simulink model "phasemixer"  (R2020a)
settings: Solver=VariableStepAuto  StartTime=0.0  StopTime=10  MaxStep=1e-3  RelTol=1e-3
InitFcn:
  | Fm = 1e9 , Tm = 1/Fm
libraries: simulink x4, msbPllFoundation x1
settings Model: Creator=hassa  LastModifiedBy=hassa

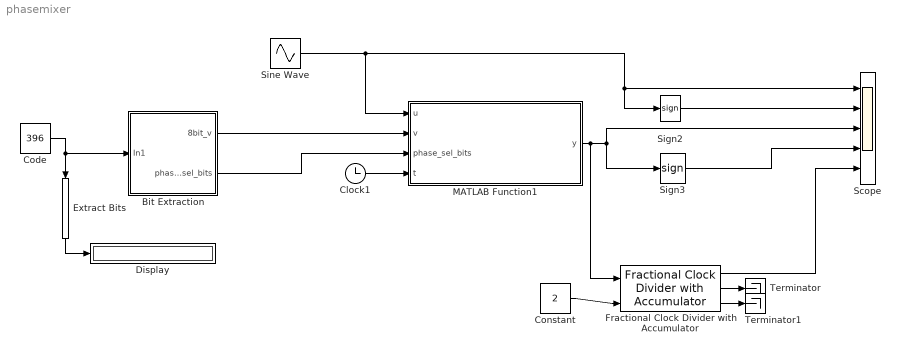
== system phasemixer ==
  Bit Extraction : Subsystem
  Clock1 : Clock
  Code : Constant  Value=396  OutDataTypeStr=uint16
  Constant : Constant  Value=2
  Display : Display
      settings: Format=binary (Stored Integer)
  Extract Bits : simulink/Logic and Bit Operations/Extract Bits  bitsToExtract=Range of bits  numBits=8  bitIdxRange=[0 9]  outScalingMode=Preserve fixed-point scaling
  Fractional Clock Divider with Accumulator : msbPllFoundation/Fractional Clock Divider with Accumulator  ExtraBuffer=on  NBuffer=1
      settings: SourceProductBaseCode=AM
  MATLAB Function1 : MATLAB Function  TreatAsAtomicUnit=on
  Scope : Scope  NumInputPorts=5
  Sign2 : Signum
  Sign3 : Signum
  Sine Wave : Sin  Frequency=2*pi  SampleTime=0
  Terminator : Terminator
  Terminator1 : Terminator
  wires:
  Code/1 -> Bit Extraction/1(In1), Extract Bits/1
  Bit Extraction/1(8bit_v) -> MATLAB Function1/2(v)
  Bit Extraction/2(phase_sel_bits) -> MATLAB Function1/3(phase_sel_bits)
  Clock1/1 -> MATLAB Function1/4(t)
  Sign2/1 -> Scope/2
  Sign3/1 -> Scope/4
  MATLAB Function1/1(y) -> Fractional Clock Divider with Accumulator/1, Scope/3, Sign3/1
  Extract Bits/1 -> Display/1
  Constant/1 -> Fractional Clock Divider with Accumulator/2
  Fractional Clock Divider with Accumulator/1 -> Scope/5
  Fractional Clock Divider with Accumulator/3 -> Terminator1/1
  Fractional Clock Divider with Accumulator/2 -> Terminator/1
  Sine Wave/1 -> MATLAB Function1/1(u), Scope/1, Sign2/1

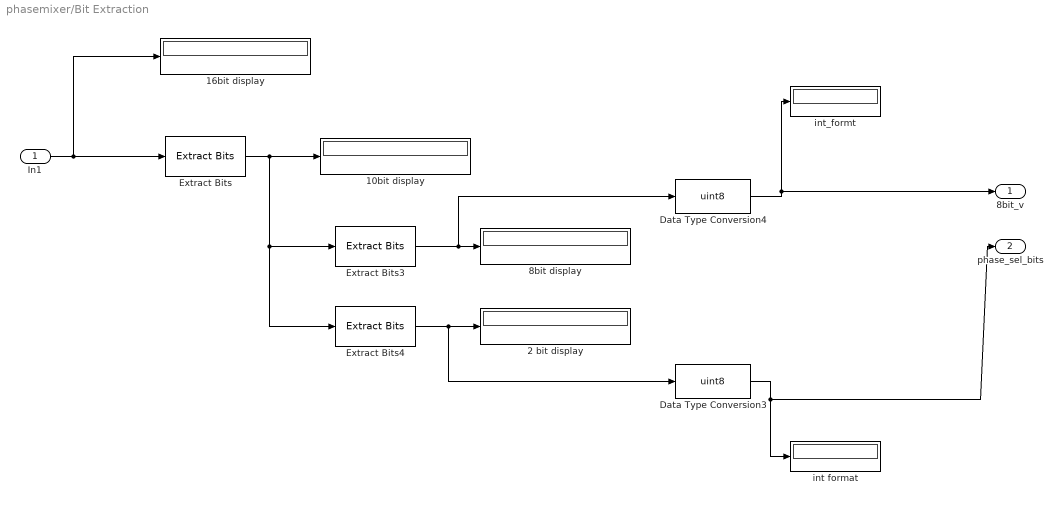
== system phasemixer/Bit Extraction ==
  In1 : Inport
  10bit display : Display
      settings: Format=binary (Stored Integer)
  16bit display : Display
      settings: Format=binary (Stored Integer)
  2 bit display : Display
      settings: Format=binary (Stored Integer)
  8bit display : Display
      settings: Format=binary (Stored Integer)
  Data Type Conversion3 : DataTypeConversion  OutDataTypeStr=uint8
  Data Type Conversion4 : DataTypeConversion  OutDataTypeStr=uint8
  Extract Bits : simulink/Logic and Bit Operations/Extract Bits  bitsToExtract=Range of bits  numBits=8  bitIdxRange=[0 9]  outScalingMode=Preserve fixed-point scaling
  Extract Bits3 : simulink/Logic and Bit Operations/Extract Bits  bitsToExtract=Range of bits  numBits=8  bitIdxRange=[0 7]  outScalingMode=Preserve fixed-point scaling
  Extract Bits4 : simulink/Logic and Bit Operations/Extract Bits  bitsToExtract=Range of bits  numBits=8  bitIdxRange=[8 9]  outScalingMode=Treat bit field as an integer
  int format : Display
  int_formt : Display
  8bit_v : Outport
  phase_sel_bits : Outport  Port=2  VectorParamsAs1DForOutWhenUnconnected=off
  wires:
  In1/1 -> Extract Bits/1, 16bit display/1
  Extract Bits4/1 -> Data Type Conversion3/1, 2 bit display/1
  Extract Bits3/1 -> Data Type Conversion4/1, 8bit display/1
  Extract Bits/1 -> Extract Bits4/1, Extract Bits3/1, 10bit display/1
  Data Type Conversion3/1 -> int format/1, phase_sel_bits/1
  Data Type Conversion4/1 -> 8bit_v/1, int_formt/1

== matlab function phasemixer/MATLAB Function1 ==
  data: u input; y output; v input; phase_sel_bits input; t input
function y  = fcn( u, v, phase_sel_bits, t)

f = 1 ;
% Initialize p1 and p2
p1 = 0.0;
p2 = 0.0;
v1 = double (v)


if phase_sel_bits == 0
    p1 = 0;
    p2 = 90;
elseif phase_sel_bits == 1
    p1 = 90;
    p2 = 180;        
elseif phase_sel_bits == 2
    p1 = 180;
    p2 = 270; 
else
    p1 = 270;
    p2 = 360;    
end

x1 = double(p2*v1)
x2 = double(p1*(255-v1))

inter_pol = (v1/ 255.0) *p2 + ((255.0 - v1) /255.0) *p1 ;
x = double(inter_pol)

fprintf('p1 = %f , p2 = %f , interpol = %f' , p1 , p2 , x)
y = sin(2*pi*t - deg2rad(x))* u

end
